simulink model "testUntilRoll_th"  (R2018b)
settings: Solver=ode3  StartTime=0.0  StopTime=sim_time  FixedStep=.001  RelTol=1e-3
values from neighbouring files (symbols this model uses):
  flow = [1.5;0;0;]    [testUntilRoll_ts.m]
  maxBank = 45*pi/180    (= 0.785398163397)    [testUntilRoll_ts.m]
undefined symbols (not defined in the file or in its folder): accelMag, init_pos, init_vel_tan, pathFollowingController_cl, setpointToOutput_cl, Subsystem, tau, tau_chi
libraries: filteredPIDController_ul x4, eulAng2RotMat_ul x2, schmehlTangentRotation_ul x2, cartToSphere_ul x1, vectorNormalizer_ul x1, angleBtw2Vecs_ul x1, vrlib x1, courseFollow_cl x1
settings Model: Creator=jldanie5  LastModifiedBy=jldanie5
settings DebuggingCC: BusObjectLabelMismatch=none

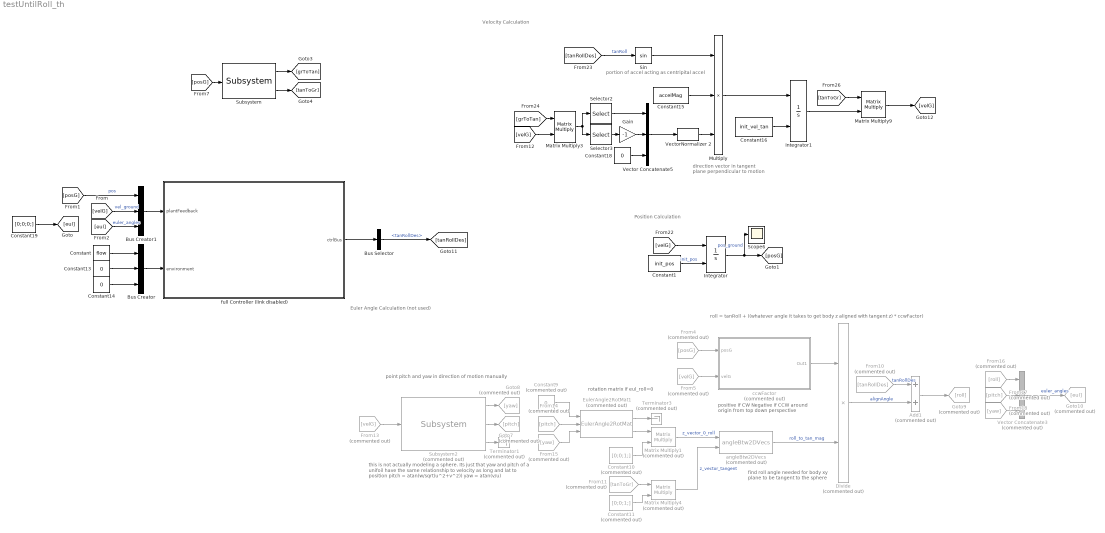
== system testUntilRoll_th ==
  note: portion of accel acting as centripital accel
  note: direction vector in tangent
      | plane perpendicular to motion
  note: find roll angle needed for body xy
      | plane to be tangent to the sphere
  note: point pitch and yaw in direction of motion manually
  note: rotation matrix if eul_roll=0
  note: Euler Angle Calculation (not used)
  note: Position Calculation
  note: Velocity Calculation
  note: this is not actually modeling a sphere.
      | Its just that yaw and pitch of a unifoil
      | have the same relationship to velocity as long and lat to position
      | pitch = atan(w/sqrt(u^2+v^2))
      | yaw = atan(v/u)
  note: roll = tanRoll + ((whatever angle it takes to get body z aligned with tangent z) * ccwFactor)
  note: positive if CW
      | Negative if CCW
      | around origin from top down perspective
  Add1 : Sum  Commented=on
  Bus Creator : BusCreator  Inputs=3  OutDataTypeStr=Bus: envBus
  Bus Creator1 : BusCreator  Inputs=3
  Bus Selector : BusSelector  OutputSignals=tanRollDes
  Constant : Constant  Value=flow
  Constant1 : Constant  Value=init_pos
  Constant10 : Constant  Commented=on  Value=[0;0;1;]
  Constant11 : Constant  Commented=on  Value=[0;0;1;]
  Constant13 : Constant  Value=0
  Constant14 : Constant  Value=0
  Constant15 : Constant  Value=accelMag
  Constant16 : Constant  Value=init_vel_tan
  Constant18 : Constant  Value=0
  Constant19 : Constant  Value=[0;0;0;]
  Constant9 : Constant  Commented=on  Value=0
  Divide : Product  Commented=on  Inputs=**
  EulerAngle2RotMat1 : eulAng2RotMat_ul/EulerAngle2RotMat  Commented=on  SystemSampleTime=-1
  From10 : From  Commented=on  GotoTag=tanRollDes
  From11 : From  Commented=on  GotoTag=tanToGr
  From13 : From  Commented=on  GotoTag=velG
  From14 : From  Commented=on  GotoTag=pitch
  From15 : From  Commented=on  GotoTag=yaw
  From16 : From  Commented=on  GotoTag=roll
  From17 : From  Commented=on  GotoTag=pitch
  From18 : From  Commented=on  GotoTag=yaw
  From4 : From  Commented=on  GotoTag=posG
  From5 : From  Commented=on  GotoTag=velG
  Gain : Gain  Gain=-1
  Goto10 : Goto  Commented=on  GotoTag=eul
  Goto7 : Goto  Commented=on  GotoTag=pitch
  Goto8 : Goto  Commented=on  GotoTag=yaw
  Goto9 : Goto  Commented=on  GotoTag=roll
  Integrator : Integrator  InitialConditionSource=external
  Integrator1 : Integrator  InitialConditionSource=external
  Matrix Multiply1 : Product  Commented=on  Multiplication=Matrix(*)
  Matrix Multiply3 : Product  Multiplication=Matrix(*)
  Matrix Multiply4 : Product  Commented=on  Multiplication=Matrix(*)
  Matrix Multiply9 : Product  Multiplication=Matrix(*)
  Multiply : Product  Inputs=3
  Scope6 : Scope
  Selector2 : Selector  InputPortWidth=3  IndexOptions=Index vector (dialog)  Indices=2  OutputSizes=1
  Selector3 : Selector  InputPortWidth=3  IndexOptions=Index vector (dialog)  Indices=1  OutputSizes=1
  Sin : Trigonometry
  Subsystem : schmehlTangentRotation_ul/Subsystem  SystemSampleTime=-1
  Subsystem2 : cartToSphere_ul/Subsystem  Commented=on  SystemSampleTime=-1
  Terminator1 : Terminator  Commented=on
  Terminator3 : Terminator  Commented=on
  Vector Concatenate3 : Concatenate  Commented=on  NumInputs=3
  Vector Concatenate5 : Concatenate  NumInputs=3
  VectorNormalizer 2 : vectorNormalizer_ul/VectorNormalizer   SystemSampleTime=-1
  angleBtw2DVecs : angleBtw2Vecs_ul/angleBtw2DVecs  Commented=on  SystemSampleTime=-1
  ccwFactor : Subsystem  Commented=on
  full Controller (link disabled) : Subsystem  AncestorBlock=pathFollowingController_cl/Subsystem  mask{a_user=1, b_user=1, phi_user=.5}
      mask prompts: a_user "Path Param A"; b_user "Path Param B"; phi_user "Path Param Phi"
  wires:
  full Controller (link disabled)/1(ctrlBus) -> Bus Selector/1
  Bus Creator/1 -> full Controller (link disabled)/2(environment)
  Constant/1 -> Bus Creator/1
  Constant1/1 -> Integrator/2  "init_pos"
  Integrator/1 -> Scope6/1, [posG]  "pos_ground"
  [posG] -> Bus Creator1/1  "pos"
  [velG] -> Bus Creator1/2  "vel_ground"
  [eul] -> Bus Creator1/3  "euler_angles"
  Bus Creator1/1 -> full Controller (link disabled)/1(plantFeedback)
  [posG] -> Subsystem/1
  Subsystem/1 -> [grToTan]
  Subsystem/2 -> [tanToGr]
  From13/1 -> Subsystem2/1
  Subsystem2/2 -> Goto7/1
  Subsystem2/1 -> Goto8/1
  Subsystem2/3 -> Terminator1/1
  From14/1 -> EulerAngle2RotMat1/2
  From15/1 -> EulerAngle2RotMat1/3
  Constant9/1 -> EulerAngle2RotMat1/1
  EulerAngle2RotMat1/2 -> Matrix Multiply1/1
  EulerAngle2RotMat1/1 -> Terminator3/1
  Constant10/1 -> Matrix Multiply1/2
  Matrix Multiply1/1 -> angleBtw2DVecs/1  "z_vector_0_roll"
  From11/1 -> Matrix Multiply4/1
  Constant11/1 -> Matrix Multiply4/2
  Matrix Multiply4/1 -> angleBtw2DVecs/2  "z_vector_tangent"
  angleBtw2DVecs/1 -> Divide/2  "roll_to_tan_mag"
  From5/1 -> ccwFactor/2(velG)
  From4/1 -> ccwFactor/1(posG)
  ccwFactor/1(Out1) -> Divide/1
  Divide/1 -> Add1/2  "alignAngle"
  Add1/1 -> Goto9/1
  Bus Selector/1 -> [tanRollDes]  "<tanRollDes>"
  From10/1 -> Add1/1  "tanRollDes"
  [velG] -> Integrator/1
  From16/1 -> Vector Concatenate3/1
  From18/1 -> Vector Concatenate3/3
  From17/1 -> Vector Concatenate3/2
  Vector Concatenate3/1 -> Goto10/1  "euler_angles"
  Constant13/1 -> Bus Creator/2
  Constant14/1 -> Bus Creator/3
  Constant15/1 -> Multiply/2
  [velG] -> Matrix Multiply3/2
  [grToTan] -> Matrix Multiply3/1
  Matrix Multiply3/1 -> Selector2/1, Selector3/1
  Selector2/1 -> Vector Concatenate5/1
  Constant16/1 -> Integrator1/2
  Constant18/1 -> Vector Concatenate5/3
  Selector3/1 -> Gain/1
  Gain/1 -> Vector Concatenate5/2
  Constant19/1 -> [eul]
  [tanRollDes] -> Sin/1  "tanRoll"
  VectorNormalizer 2/1 -> Multiply/3
  Vector Concatenate5/1 -> VectorNormalizer 2/1
  Sin/1 -> Multiply/1
  Multiply/1 -> Integrator1/1
  Integrator1/1 -> Matrix Multiply9/2
  [tanToGr] -> Matrix Multiply9/1
  Matrix Multiply9/1 -> [velG]

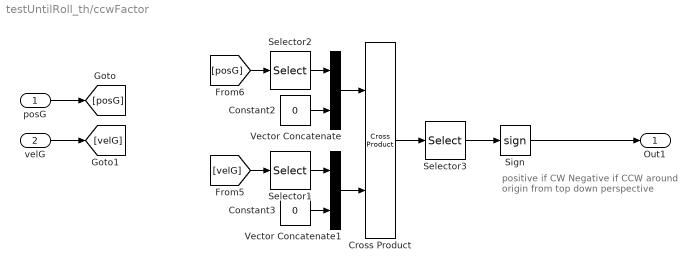
== system testUntilRoll_th/ccwFactor ==
  note: positive if CW
      | Negative if CCW
      | around origin from top down perspective
  posG : Inport
  velG : Inport  Port=2
  Constant2 : Constant  Value=0
  Constant3 : Constant  Value=0
  Cross Product : vrlib/Utilities/Cross Product
      settings: SourceProductBaseCode=VR
  Selector1 : Selector  InputPortWidth=3  IndexOptions=Index vector (dialog)  Indices=[1 2]  OutputSizes=1
  Selector2 : Selector  InputPortWidth=3  IndexOptions=Index vector (dialog)  Indices=[1 2]  OutputSizes=1
  Selector3 : Selector  InputPortWidth=3  IndexOptions=Index vector (dialog)  Indices=3  OutputSizes=1
  Sign : Signum
  Vector Concatenate : Concatenate
  Vector Concatenate1 : Concatenate
  Out1 : Outport
  wires:
  Sign/1 -> Out1/1
  Vector Concatenate1/1 -> Cross Product/2
  Vector Concatenate/1 -> Cross Product/1
  [posG] -> Selector2/1
  Selector1/1 -> Vector Concatenate1/1
  [velG] -> Selector1/1
  Selector2/1 -> Vector Concatenate/1
  Constant2/1 -> Vector Concatenate/2
  Constant3/1 -> Vector Concatenate1/2
  Selector3/1 -> Sign/1
  Cross Product/1 -> Selector3/1
  posG/1 -> [posG]
  velG/1 -> [velG]

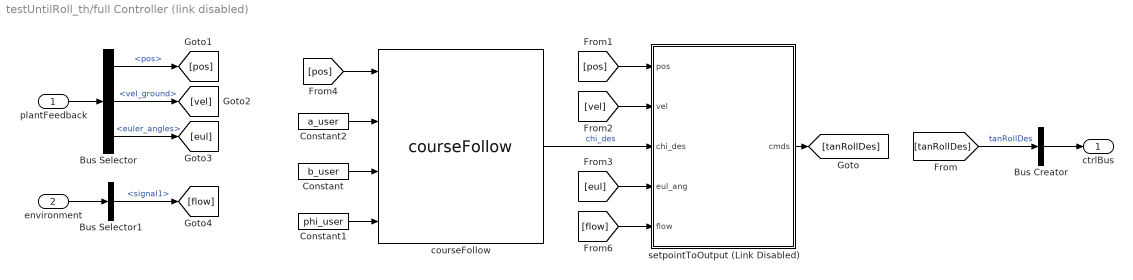
== system testUntilRoll_th/full Controller (link disabled) ==
  plantFeedback : Inport  OutDataTypeStr=Bus: plantBus
  environment : Inport  Port=2  OutDataTypeStr=Bus: envBus
  Bus Creator : BusCreator  Inputs=1  OutDataTypeStr=Bus: ctrlBus
  Bus Selector : BusSelector  OutputSignals=pos,vel_ground,euler_angles
  Bus Selector1 : BusSelector  OutputSignals=signal1
  Constant : Constant  Value=b_user
  Constant1 : Constant  Value=phi_user
  Constant2 : Constant  Value=a_user
  courseFollow : courseFollow_cl/courseFollow  SystemSampleTime=-1
      link override chiMachine: error_upper_lim=3*pi/180
  setpointToOutput (Link Disabled) : Subsystem  AncestorBlock=setpointToOutput_cl/Subsystem  mask{maxBank=maxBank, AoA_des=0, controlMat=0, ctrlSigMax=0}
      mask prompts: maxBank "Maximum Bank Angle"; AoA_des "Desired Angle of Attack"; controlMat "Matrix to convert Desired Moments to Control Signals"; ctrlSigMax "Max control signal"
  ctrlBus : Outport
  wires:
  [flow] -> setpointToOutput (Link Disabled)/5(flow)
  Bus Selector1/1 -> [flow]  "<signal1>"
  Constant1/1 -> courseFollow/4
  Constant/1 -> courseFollow/3
  Constant2/1 -> courseFollow/2
  [pos] -> courseFollow/1
  [tanRollDes] -> Bus Creator/1  "tanRollDes"
  [eul] -> setpointToOutput (Link Disabled)/4(eul_ang)
  [vel] -> setpointToOutput (Link Disabled)/2(vel)
  [pos] -> setpointToOutput (Link Disabled)/1(pos)
  Bus Selector/3 -> [eul]  "<euler_angles>"
  Bus Selector/1 -> [pos]  "<pos>"
  Bus Selector/2 -> [vel]  "<vel_ground>"
  plantFeedback/1 -> Bus Selector/1
  environment/1 -> Bus Selector1/1
  Bus Creator/1 -> ctrlBus/1
  courseFollow/1 -> setpointToOutput (Link Disabled)/3(chi_des)  "chi_des"
  setpointToOutput (Link Disabled)/1(cmds) -> [tanRollDes]

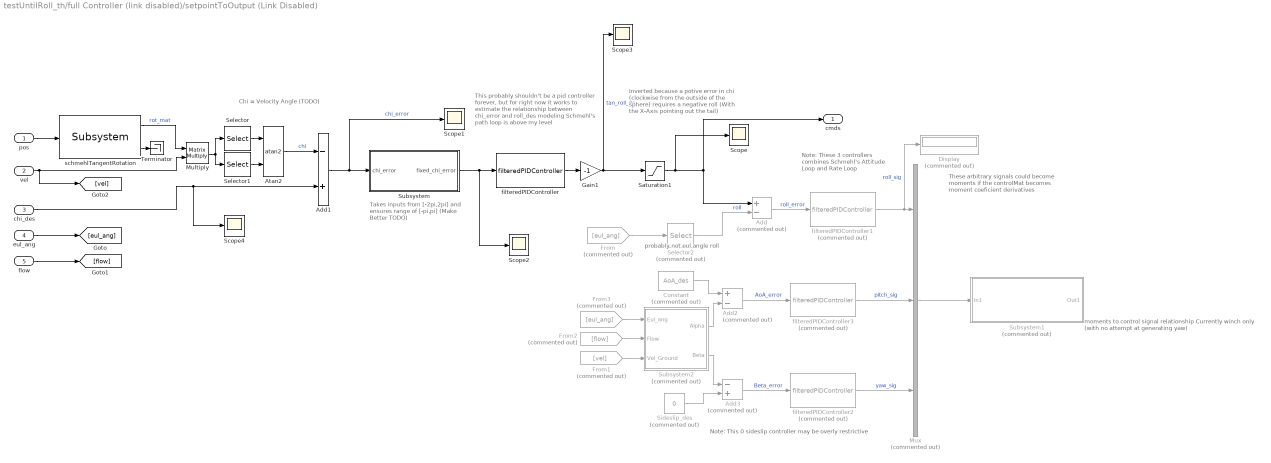
== system testUntilRoll_th/full Controller (link disabled)/setpointToOutput (Link Disabled) ==
  note: moments to control signal relationship
      | Currently winch only (with no attempt at generating yaw)
  note: Takes inputs from [-2pi,2pi] and
      | ensures range of [-pi,pi]
      | (Make Better TODO)
  note: This probably shouldn't be a pid
      | controller forever, but for right now
      | it works to estimate the relationship
      | between chi_error and roll_des
      |
      | modeling Schmehl's path loop is above
      | my level
  note: Note: This 0 sideslip controller may be overly restrictive
  note: Note: These 3 controllers
      | combines Schmehl's Attitude
      | Loop and Rate Loop
  note: Inverted because a potive error
      | in chi (clockwise from the outside of
      | the sphere) requires a negative roll
      | (With the X-Axis pointing out the tail)
  note: These arbitrary signals could become
      | moments if the controlMat
      | becomes moment coeficient derivatives
  note: Chi = Velocity Angle (TODO)
  note: probably not eul angle roll
  pos : Inport
  vel : Inport  Port=2
  chi_des : Inport  Port=3
  eul_ang : Inport  Port=4
  flow : Inport  Port=5
  Add : Sum  Commented=on  Inputs=+-
  Add1 : Sum  Inputs=-+
  Add2 : Sum  Commented=on  Inputs=+-
  Add3 : Sum  Commented=on  Inputs=-+
  Atan2 : Trigonometry  Operator=atan2
  Constant : Constant  Commented=on  Value=AoA_des
  Display : Display  Commented=on
  From : From  Commented=on  GotoTag=eul_ang
  From1 : From  Commented=on  GotoTag=vel
  From2 : From  Commented=on  GotoTag=flow
  From3 : From  Commented=on  GotoTag=eul_ang
  Gain1 : Gain  Gain=-1
  Multiply : Product  Multiplication=Matrix(*)
  Mux : Mux  Commented=on  Inputs=3
  Saturation1 : Saturate  UpperLimit=maxBank  LowerLimit=-maxBank
  Scope{,1..4} (5 alike) : Scope
  Selector : Selector  InputPortWidth=3  IndexOptions=Index vector (dialog)  Indices=2  OutputSizes=1
  Selector1 : Selector  InputPortWidth=3  IndexOptions=Index vector (dialog)  Indices=1  OutputSizes=1
  Selector2 : Selector  Commented=on  InputPortWidth=3  IndexOptions=Index vector (dialog)  Indices=1  OutputSizes=1
  Sideslip_des : Constant  Commented=on  Value=0
  Subsystem : Subsystem
  Subsystem1 : Subsystem  Commented=on
  Subsystem2 : Subsystem  Commented=on
  Terminator : Terminator
  filteredPIDController : filteredPIDController_ul/filteredPIDController  kp=kp_chi  ki=ki_chi  kd=kd_chi  Value=tau_chi
  filteredPIDController1 : filteredPIDController_ul/filteredPIDController  Commented=on  kp=kp_L  ki=0  kd=kd_L  Value=tau
  filteredPIDController2 : filteredPIDController_ul/filteredPIDController  Commented=on  kp=kp_L  ki=0  kd=kd_L  Value=tau
  filteredPIDController3 : filteredPIDController_ul/filteredPIDController  Commented=on  kp=kp_M  ki=0  kd=kd_M  Value=tau
  schmehlTangentRotation : schmehlTangentRotation_ul/Subsystem  SystemSampleTime=-1
  cmds : Outport
  wires:
  Mux/1 -> Subsystem1/1(In1)
  Saturation1/1 -> Scope/1, Add/1, cmds/1
  Gain1/1 -> Scope3/1, Saturation1/1  "tan_roll_des"
  Add3/1 -> filteredPIDController2/1  "Beta_error"
  Sideslip_des/1 -> Add3/2
  Subsystem2/2(Beta) -> Add3/1
  Add2/1 -> filteredPIDController3/1  "AoA_error"
  Constant/1 -> Add2/1
  Subsystem2/1(Alpha) -> Add2/2
  From1/1 -> Subsystem2/3(Vel_Ground)
  From2/1 -> Subsystem2/2(Flow)
  From3/1 -> Subsystem2/1(Eul_ang)
  filteredPIDController3/1 -> Mux/2  "pitch_sig"
  filteredPIDController2/1 -> Mux/3  "yaw_sig"
  filteredPIDController/1 -> Gain1/1
  Add1/1 -> Subsystem/1(chi_error), Scope1/1  "chi_error"
  flow/1 -> [flow]
  eul_ang/1 -> [eul_ang]
  filteredPIDController1/1 -> Mux/1, Display/1  "roll_sig"
  Add/1 -> filteredPIDController1/1  "roll_error"
  Selector2/1 -> Add/2  "roll"
  From/1 -> Selector2/1
  chi_des/1 -> Scope4/1, Add1/2
  Atan2/1 -> Add1/1  "chi"
  Selector/1 -> Atan2/1
  Selector1/1 -> Atan2/2
  Multiply/1 -> Selector1/1, Selector/1
  vel/1 -> [vel], Multiply/2
  pos/1 -> schmehlTangentRotation/1
  schmehlTangentRotation/1 -> Multiply/1  "rot_mat"
  schmehlTangentRotation/2 -> Terminator/1
  Subsystem/1(fixed_chi_error) -> Scope2/1, filteredPIDController/1

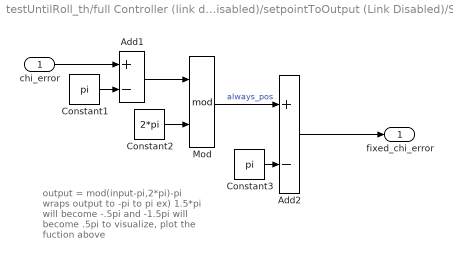
== system testUntilRoll_th/full Controller (link disabled)/setpointToOutput (Link Disabled)/Subsystem ==
  note: output = mod(input-pi,2*pi)-pi
      | wraps output to -pi to pi
      |
      | ex) 1.5*pi will become -.5pi
      | 	and -1.5pi will become .5pi
      |
      | to visualize, plot the fuction above
  chi_error : Inport
  Add1 : Sum  Inputs=+-
  Add2 : Sum  Inputs=+-
  Constant1 : Constant  Value=pi
  Constant2 : Constant  Value=2*pi
  Constant3 : Constant  Value=pi
  Mod : Math  Operator=mod  SaturateOnIntegerOverflow=on
  fixed_chi_error : Outport
  wires:
  Constant3/1 -> Add2/2
  chi_error/1 -> Add1/1
  Add1/1 -> Mod/1
  Mod/1 -> Add2/1  "always_pos"
  Add2/1 -> fixed_chi_error/1
  Constant1/1 -> Add1/2
  Constant2/1 -> Mod/2

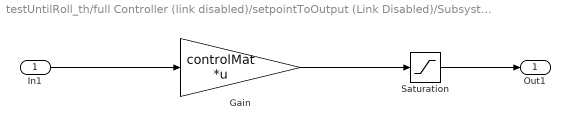
== system testUntilRoll_th/full Controller (link disabled)/setpointToOutput (Link Disabled)/Subsystem1 ==
  In1 : Inport
  Gain : Gain  Gain=controlMat  Multiplication=Matrix(K*u)
  Saturation : Saturate  UpperLimit=ctrlSigMax  LowerLimit=-ctrlSigMax
  Out1 : Outport
  wires:
  Saturation/1 -> Out1/1
  In1/1 -> Gain/1
  Gain/1 -> Saturation/1

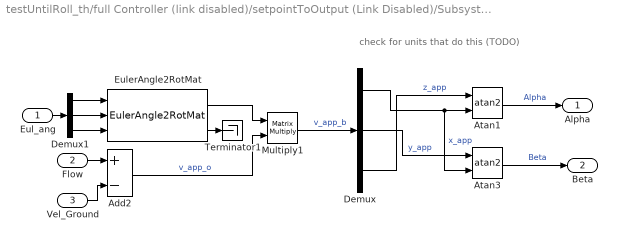
== system testUntilRoll_th/full Controller (link disabled)/setpointToOutput (Link Disabled)/Subsystem2 ==
  note: check for units that do this (TODO)
  Eul_ang : Inport
  Flow : Inport  Port=2
  Vel_Ground : Inport  Port=3
  Add2 : Sum  Inputs=+-
  Atan1 : Trigonometry  Operator=atan2
  Atan3 : Trigonometry  Operator=atan2
  Demux : Demux  Outputs=3
  Demux1 : Demux  Outputs=3
  EulerAngle2RotMat : eulAng2RotMat_ul/EulerAngle2RotMat  SystemSampleTime=-1
  Multiply1 : Product  Multiplication=Matrix(*)
  Terminator1 : Terminator
  Alpha : Outport
  Beta : Outport  Port=2
  wires:
  Demux1/1 -> EulerAngle2RotMat/1
  Demux1/2 -> EulerAngle2RotMat/2
  Demux1/3 -> EulerAngle2RotMat/3
  Vel_Ground/1 -> Add2/2
  Atan1/1 -> Alpha/1  "Alpha"
  Flow/1 -> Add2/1
  Atan3/1 -> Beta/1  "Beta"
  Add2/1 -> Multiply1/2  "v_app_o"
  Eul_ang/1 -> Demux1/1
  Multiply1/1 -> Demux/1  "v_app_b"
  EulerAngle2RotMat/1 -> Multiply1/1
  Demux/2 -> Atan3/1  "y_app"
  Demux/3 -> Atan1/1  "z_app"
  EulerAngle2RotMat/2 -> Terminator1/1
  Demux/1 -> Atan3/2, Atan1/2  "x_app"
